simulink model "stint_mdl"  (R2021b)
settings: Solver=ode1  StartTime=0.0  StopTime=7  FixedStep=0.0001  MaxStep=0.1  MinStep=0.001  RelTol=1e-3
values from neighbouring files (symbols this model uses):
  A = [0 1; 0 0]    [pendulum_data.m]
  B = [0;1]    [pendulum_data.m]
  C = C([1,3],:)    [comp_data.m]    (also in pendulum_data.m = [1 1])
  Gamma = diag([-0.5])    [obsint_data.m]    (also in stmod_data.m = diag([-0.025]))
  L = -inv(S*B)*(S*Am-Phi*S)    [stmod_data.m]
  rho = 1    [comp_data.m]    (also in obsint_data.m; obsmod_data.m; outmod_data.m; outmodc_data.m)
  S = rpp(A,B,psm)    [obsint_data.m]    (also in stint_data.m = rpp(A,B,sp); stmod_data.m = inv(S*B)*S; streg_data.m = rpp(A,B,sp))
undefined symbols (not defined in the file or in its folder): Lam, Lr, Lrdot, m, n, P, p, Sr
settings Model: Creator=w.schwamm  LastModifiedBy=w.schwamm
settings DataIOCC: SaveOutput=off  SaveTime=off  ReturnWorkspaceOutputs=off  StateSaveName=x  TimeSaveName=t  OutputSaveName=y

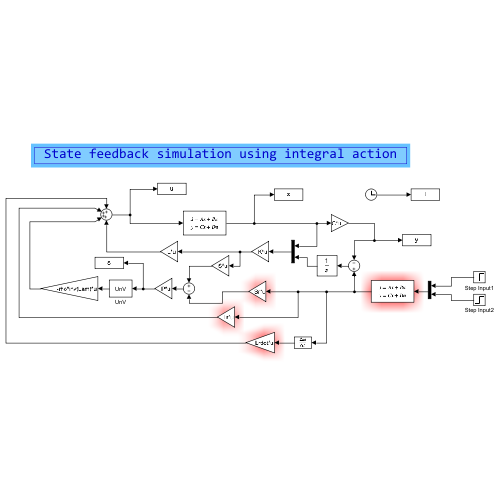
[thumbnail: Simulink's stored preview of the top-level diagram]
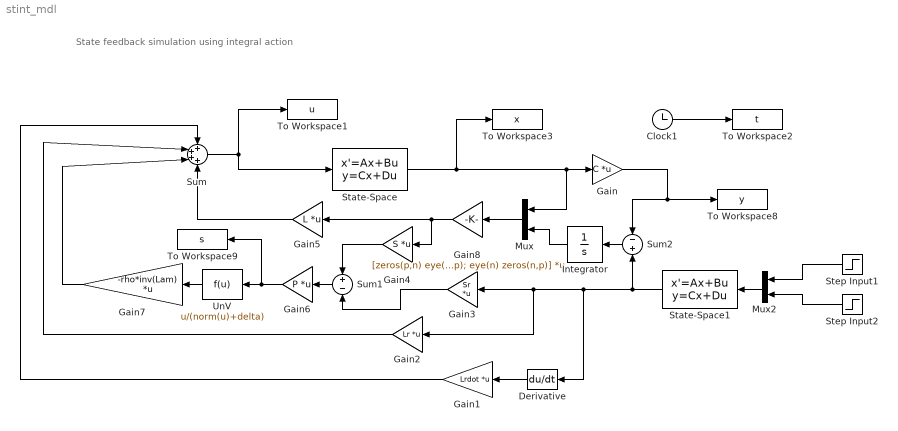
== system stint_mdl ==
  note: State feedback simulation using integral action
  Clock1 : Clock
  Derivative : Derivative
  Gain : Gain  Gain=C  Multiplication=Matrix(K*u)
  Gain1 : Gain  Gain=Lrdot  Multiplication=Matrix(K*u)
  Gain2 : Gain  Gain=Lr  Multiplication=Matrix(K*u)
  Gain3 : Gain  Gain=Sr  Multiplication=Matrix(K*u)
  Gain4 : Gain  Gain=S  Multiplication=Matrix(K*u)
  Gain5 : Gain  Gain=L  Multiplication=Matrix(K*u)
  Gain6 : Gain  Gain=P  Multiplication=Matrix(K*u)
  Gain7 : Gain  Gain=-rho*inv(Lam)  Multiplication=Matrix(K*u)
  Gain8 : Gain  Gain=[zeros(p,n) eye(p); eye(n) zeros(n,p)]  Multiplication=Matrix(K*u)
  Integrator : Integrator
  Mux : Mux  Inputs=2
  Mux2 : Mux  Inputs=2
  State-Space : StateSpace  A=A  B=B  C=eye(n)  D=zeros(n,m)  InitialCondition=0
  State-Space1 : StateSpace  A=Gamma  B=Gamma  C=-eye(p)  D=zeros(p,p)  InitialCondition=0
  Step Input1 : Step  Time=0  After=0  SampleTime=0
  Step Input2 : Step  Time=0  SampleTime=0
  Sum : Sum  Inputs=++++
  Sum1 : Sum  Inputs=+-
  Sum2 : Sum  Inputs=-+
  To Workspace1 : ToWorkspace  VariableName=u  SaveFormat=Timeseries  SampleTime=-1
      settings: MaxDataPoints=1000000
  To Workspace2 : ToWorkspace  VariableName=t  SaveFormat=Timeseries  SampleTime=-1
      settings: MaxDataPoints=1000000
  To Workspace3 : ToWorkspace  VariableName=x  SaveFormat=Timeseries  SampleTime=-1
      settings: MaxDataPoints=1000000
  To Workspace8 : ToWorkspace  VariableName=y  SaveFormat=Timeseries  SampleTime=-1
      settings: MaxDataPoints=1000000
  To Workspace9 : ToWorkspace  VariableName=s  SaveFormat=Timeseries  SampleTime=-1
      settings: MaxDataPoints=1000000
  UnV : Fcn  Expr=u/(norm(u)+delta)  mask(unit vector){delta=0.001}
      mask Display: disp('UnV')
  wires:
  Clock1/1 -> To Workspace2/1
  UnV/1 -> Gain7/1
  Gain6/1 -> UnV/1, To Workspace9/1
  Gain1/1 -> Sum/1
  Sum/1 -> State-Space/1, To Workspace1/1
  Sum1/1 -> Gain6/1
  Gain4/1 -> Sum1/1
  Gain3/1 -> Sum1/2
  Gain7/1 -> Sum/3
  Gain5/1 -> Sum/4
  Sum2/1 -> Integrator/1
  State-Space1/1 -> Gain3/1, Gain2/1, Derivative/1, Sum2/2
  Derivative/1 -> Gain1/1
  Gain2/1 -> Sum/2
  Mux2/1 -> State-Space1/1
  Step Input1/1 -> Mux2/1
  Step Input2/1 -> Mux2/2
  Mux/1 -> Gain8/1
  Gain8/1 -> Gain5/1, Gain4/1
  Integrator/1 -> Mux/2
  State-Space/1 -> Gain/1, Mux/1, To Workspace3/1
  Gain/1 -> Sum2/1, To Workspace8/1
